simulink model "CEN598_HW2"  (R2015b)
settings: Solver=FixedStepDiscrete  SolverMode=SingleTasking  StartTime=0.0  StopTime=2.5e-6  RelTol=1e-3
libraries: shlslibv1 x212
(part 1 of 2)
settings Model: synDspstartup=OK  Creator=amitra5  LastModifiedBy=sjparekh
settings DataIOCC: SaveFormat=Array  SaveOutput=off  SignalLogging=off  SaveTime=off
settings OptimizationCC: DefaultParameterBehavior=Inlined
settings DebuggingCC: AlgebraicLoopMsg=error  SolverPrmCheckMsg=warning  InheritedTsInSrcMsg=none
settings HardwareCC: ProdBitPerPointer=32  ProdLargestAtomicFloat=None  ProdIntDivRoundTo=Undefined  ProdEndianess=Unspecified  ProdWordSize=32  ProdHWDeviceType=32-bit Generic
settings GRTTargetCC: GeneratePreprocessorConditionals=Disable all
settings ConfigComp: CovModelRefEnable=Off  CovSFcnEnable=off

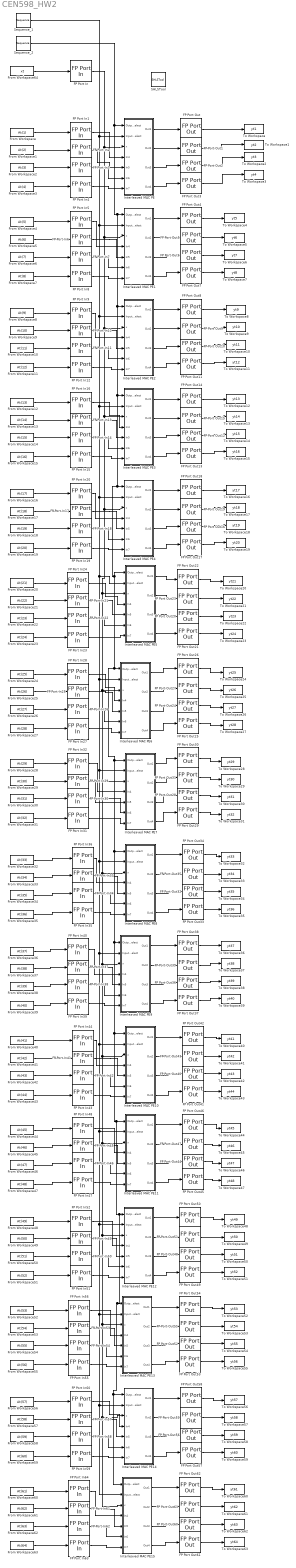
== system CEN598_HW2 ==
  FP Port In{,1..64} (65 alike) : shlslibv1/Floating Point/FP Port In  synBlockType=custom  synLatency=1  syn_exp_wl=11  syn_frac_wl=52  syn_out_st=1/284.04e6  syn_capture=on  syn_register=on  syn_opt_ports=off
  FP Port Out{,1..63} (64 alike) : shlslibv1/Floating Point/FP Port Out  synBlockType=custom  synLatency=1  syn_exp_wl=11  syn_frac_wl=52  syn_capture=on  syn_register=on
  From Workspace : FromWorkspace  VariableName=At(1)  Interpolate=off  OutputAfterFinalValue=Holding final value
  From Workspace1 : FromWorkspace  VariableName=At(2)  Interpolate=off  OutputAfterFinalValue=Holding final value
  From Workspace10 : FromWorkspace  VariableName=At(11)  Interpolate=off  OutputAfterFinalValue=Holding final value
  From Workspace11 : FromWorkspace  VariableName=At(12)  Interpolate=off  OutputAfterFinalValue=Holding final value
  From Workspace12 : FromWorkspace  VariableName=At(13)  Interpolate=off  OutputAfterFinalValue=Holding final value
  From Workspace13 : FromWorkspace  VariableName=At(14)  Interpolate=off  OutputAfterFinalValue=Holding final value
  From Workspace14 : FromWorkspace  VariableName=At(15)  Interpolate=off  OutputAfterFinalValue=Holding final value
  From Workspace15 : FromWorkspace  VariableName=At(16)  Interpolate=off  OutputAfterFinalValue=Holding final value
  From Workspace16 : FromWorkspace  VariableName=At(17)  Interpolate=off  OutputAfterFinalValue=Holding final value
  From Workspace17 : FromWorkspace  VariableName=At(18)  Interpolate=off  OutputAfterFinalValue=Holding final value
  From Workspace18 : FromWorkspace  VariableName=At(19)  Interpolate=off  OutputAfterFinalValue=Holding final value
  From Workspace19 : FromWorkspace  VariableName=At(20)  Interpolate=off  OutputAfterFinalValue=Holding final value
  From Workspace2 : FromWorkspace  VariableName=At(3)  Interpolate=off  OutputAfterFinalValue=Holding final value
  From Workspace20 : FromWorkspace  VariableName=At(21)  Interpolate=off  OutputAfterFinalValue=Holding final value
  From Workspace21 : FromWorkspace  VariableName=At(22)  Interpolate=off  OutputAfterFinalValue=Holding final value
  From Workspace22 : FromWorkspace  VariableName=At(23)  Interpolate=off  OutputAfterFinalValue=Holding final value
  From Workspace23 : FromWorkspace  VariableName=At(24)  Interpolate=off  OutputAfterFinalValue=Holding final value
  From Workspace24 : FromWorkspace  VariableName=At(25)  Interpolate=off  OutputAfterFinalValue=Holding final value
  From Workspace25 : FromWorkspace  VariableName=At(26)  Interpolate=off  OutputAfterFinalValue=Holding final value
  From Workspace26 : FromWorkspace  VariableName=At(27)  Interpolate=off  OutputAfterFinalValue=Holding final value
  From Workspace27 : FromWorkspace  VariableName=At(28)  Interpolate=off  OutputAfterFinalValue=Holding final value
  From Workspace28 : FromWorkspace  VariableName=At(29)  Interpolate=off  OutputAfterFinalValue=Holding final value
  From Workspace29 : FromWorkspace  VariableName=At(30)  Interpolate=off  OutputAfterFinalValue=Holding final value
  From Workspace3 : FromWorkspace  VariableName=At(4)  Interpolate=off  OutputAfterFinalValue=Holding final value
  From Workspace30 : FromWorkspace  VariableName=At(31)  Interpolate=off  OutputAfterFinalValue=Holding final value
  From Workspace31 : FromWorkspace  VariableName=At(32)  Interpolate=off  OutputAfterFinalValue=Holding final value
  From Workspace32 : FromWorkspace  VariableName=At(33)  Interpolate=off  OutputAfterFinalValue=Holding final value
  From Workspace33 : FromWorkspace  VariableName=At(34)  Interpolate=off  OutputAfterFinalValue=Holding final value
  From Workspace34 : FromWorkspace  VariableName=At(35)  Interpolate=off  OutputAfterFinalValue=Holding final value
  From Workspace35 : FromWorkspace  VariableName=At(36)  Interpolate=off  OutputAfterFinalValue=Holding final value
  From Workspace36 : FromWorkspace  VariableName=At(37)  Interpolate=off  OutputAfterFinalValue=Holding final value
  From Workspace37 : FromWorkspace  VariableName=At(38)  Interpolate=off  OutputAfterFinalValue=Holding final value
  From Workspace38 : FromWorkspace  VariableName=At(39)  Interpolate=off  OutputAfterFinalValue=Holding final value
  From Workspace39 : FromWorkspace  VariableName=At(40)  Interpolate=off  OutputAfterFinalValue=Holding final value
  From Workspace4 : FromWorkspace  VariableName=At(5)  Interpolate=off  OutputAfterFinalValue=Holding final value
  From Workspace40 : FromWorkspace  VariableName=At(41)  Interpolate=off  OutputAfterFinalValue=Holding final value
  From Workspace41 : FromWorkspace  VariableName=At(42)  Interpolate=off  OutputAfterFinalValue=Holding final value
  From Workspace42 : FromWorkspace  VariableName=At(43)  Interpolate=off  OutputAfterFinalValue=Holding final value
  From Workspace43 : FromWorkspace  VariableName=At(44)  Interpolate=off  OutputAfterFinalValue=Holding final value
  From Workspace44 : FromWorkspace  VariableName=At(45)  Interpolate=off  OutputAfterFinalValue=Holding final value
  From Workspace45 : FromWorkspace  VariableName=At(46)  Interpolate=off  OutputAfterFinalValue=Holding final value
  From Workspace46 : FromWorkspace  VariableName=At(47)  Interpolate=off  OutputAfterFinalValue=Holding final value
  From Workspace47 : FromWorkspace  VariableName=At(48)  Interpolate=off  OutputAfterFinalValue=Holding final value
  From Workspace48 : FromWorkspace  VariableName=At(49)  Interpolate=off  OutputAfterFinalValue=Holding final value
  From Workspace49 : FromWorkspace  VariableName=At(50)  Interpolate=off  OutputAfterFinalValue=Holding final value
  From Workspace5 : FromWorkspace  VariableName=At(6)  Interpolate=off  OutputAfterFinalValue=Holding final value
  From Workspace50 : FromWorkspace  VariableName=At(51)  Interpolate=off  OutputAfterFinalValue=Holding final value
  From Workspace51 : FromWorkspace  VariableName=At(52)  Interpolate=off  OutputAfterFinalValue=Holding final value
  From Workspace52 : FromWorkspace  VariableName=At(53)  Interpolate=off  OutputAfterFinalValue=Holding final value
  From Workspace53 : FromWorkspace  VariableName=At(54)  Interpolate=off  OutputAfterFinalValue=Holding final value
  From Workspace54 : FromWorkspace  VariableName=At(55)  Interpolate=off  OutputAfterFinalValue=Holding final value
  From Workspace55 : FromWorkspace  VariableName=At(56)  Interpolate=off  OutputAfterFinalValue=Holding final value
  From Workspace56 : FromWorkspace  VariableName=At(57)  Interpolate=off  OutputAfterFinalValue=Holding final value
  From Workspace57 : FromWorkspace  VariableName=At(58)  Interpolate=off  OutputAfterFinalValue=Holding final value
  From Workspace58 : FromWorkspace  VariableName=At(59)  Interpolate=off  OutputAfterFinalValue=Holding final value
  From Workspace59 : FromWorkspace  VariableName=At(60)  Interpolate=off  OutputAfterFinalValue=Holding final value
  From Workspace6 : FromWorkspace  VariableName=At(7)  Interpolate=off  OutputAfterFinalValue=Holding final value
  From Workspace60 : FromWorkspace  VariableName=At(61)  Interpolate=off  OutputAfterFinalValue=Holding final value
  From Workspace61 : FromWorkspace  VariableName=At(62)  Interpolate=off  OutputAfterFinalValue=Holding final value
  From Workspace62 : FromWorkspace  VariableName=At(63)  Interpolate=off  OutputAfterFinalValue=Holding final value
  From Workspace63 : FromWorkspace  VariableName=At(64)  Interpolate=off  OutputAfterFinalValue=Holding final value
  From Workspace64 : FromWorkspace  VariableName=xt  Interpolate=off  OutputAfterFinalValue=Holding final value
  From Workspace7 : FromWorkspace  VariableName=At(8)  Interpolate=off  OutputAfterFinalValue=Holding final value
  From Workspace8 : FromWorkspace  VariableName=At(9)  Interpolate=off  OutputAfterFinalValue=Holding final value
  From Workspace9 : FromWorkspace  VariableName=At(10)  Interpolate=off  OutputAfterFinalValue=Holding final value
  Interleaved MAC PE : Subsystem
  Interleaved MAC PE1 : Subsystem
  Interleaved MAC PE10 : Subsystem
  Interleaved MAC PE11 : Subsystem
  Interleaved MAC PE12 : Subsystem
  Interleaved MAC PE13 : Subsystem
  Interleaved MAC PE14 : Subsystem
  Interleaved MAC PE15 : Subsystem
  Interleaved MAC PE2 : Subsystem
  Interleaved MAC PE3 : Subsystem
  Interleaved MAC PE4 : Subsystem
  Interleaved MAC PE5 : Subsystem
  Interleaved MAC PE6 : Subsystem
  Interleaved MAC PE7 : Subsystem
  Interleaved MAC PE8 : Subsystem
  Interleaved MAC PE9 : Subsystem
  SHLSTool : shlslibv1/SHLSTool  synBlockType=tool  syn_dsp_mode=FPGA
  Sequence_1 : shlslibv1/Sources/Sequence  syn_seq_vec=[0 1 2 3 0 0 0 0 0]  syn_seq_wl=2  syn_seq_fl=0  syn_seq_dt=unsigned  syn_rst_port=off  syn_en_port=off  syn_seq_st=1/284.04e6  synBlockType=custom  synLatency=1
  Sequence_2 : shlslibv1/Sources/Sequence  syn_seq_vec=[0 0 0 0 1 2 3 0 0]  syn_seq_wl=2  syn_seq_fl=0  syn_seq_dt=unsigned  syn_rst_port=off  syn_en_port=off  syn_seq_st=1/284.04e6  synBlockType=custom  synLatency=1
  To Workspace : ToWorkspace  VariableName=yt1  SaveFormat=Structure With Time  SampleTime=-1
      settings: Save2DSignal=2-D array (concatenate along first dimension)
  To Workspace1 : ToWorkspace  VariableName=yt2  SaveFormat=Structure With Time  SampleTime=-1
      settings: Save2DSignal=2-D array (concatenate along first dimension)
  To Workspace10 : ToWorkspace  VariableName=yt11  SaveFormat=Structure With Time  SampleTime=-1
      settings: Save2DSignal=2-D array (concatenate along first dimension)
  To Workspace11 : ToWorkspace  VariableName=yt12  SaveFormat=Structure With Time  SampleTime=-1
  To Workspace12 : ToWorkspace  VariableName=yt13  SaveFormat=Structure With Time  SampleTime=-1
      settings: Save2DSignal=2-D array (concatenate along first dimension)
  To Workspace13 : ToWorkspace  VariableName=yt14  SaveFormat=Structure With Time  SampleTime=-1
      settings: Save2DSignal=2-D array (concatenate along first dimension)
  To Workspace14 : ToWorkspace  VariableName=yt15  SaveFormat=Structure With Time  SampleTime=-1
      settings: Save2DSignal=2-D array (concatenate along first dimension)
  To Workspace15 : ToWorkspace  VariableName=yt16  SaveFormat=Structure With Time  SampleTime=-1
  To Workspace16 : ToWorkspace  VariableName=yt17  SaveFormat=Structure With Time  SampleTime=-1
      settings: Save2DSignal=2-D array (concatenate along first dimension)
  To Workspace17 : ToWorkspace  VariableName=yt18  SaveFormat=Structure With Time  SampleTime=-1
      settings: Save2DSignal=2-D array (concatenate along first dimension)
  To Workspace18 : ToWorkspace  VariableName=yt19  SaveFormat=Structure With Time  SampleTime=-1
      settings: Save2DSignal=2-D array (concatenate along first dimension)
  To Workspace19 : ToWorkspace  VariableName=yt20  SaveFormat=Structure With Time  SampleTime=-1
  To Workspace2 : ToWorkspace  VariableName=yt3  SaveFormat=Structure With Time  SampleTime=-1
      settings: Save2DSignal=2-D array (concatenate along first dimension)
  To Workspace20 : ToWorkspace  VariableName=yt21  SaveFormat=Structure With Time  SampleTime=-1
      settings: Save2DSignal=2-D array (concatenate along first dimension)
  To Workspace21 : ToWorkspace  VariableName=yt22  SaveFormat=Structure With Time  SampleTime=-1
      settings: Save2DSignal=2-D array (concatenate along first dimension)
  To Workspace22 : ToWorkspace  VariableName=yt23  SaveFormat=Structure With Time  SampleTime=-1
      settings: Save2DSignal=2-D array (concatenate along first dimension)
  To Workspace23 : ToWorkspace  VariableName=yt24  SaveFormat=Structure With Time  SampleTime=-1
  To Workspace24 : ToWorkspace  VariableName=yt25  SaveFormat=Structure With Time  SampleTime=-1
      settings: Save2DSignal=2-D array (concatenate along first dimension)
  To Workspace25 : ToWorkspace  VariableName=yt26  SaveFormat=Structure With Time  SampleTime=-1
      settings: Save2DSignal=2-D array (concatenate along first dimension)
  To Workspace26 : ToWorkspace  VariableName=yt27  SaveFormat=Structure With Time  SampleTime=-1
      settings: Save2DSignal=2-D array (concatenate along first dimension)
  To Workspace27 : ToWorkspace  VariableName=yt28  SaveFormat=Structure With Time  SampleTime=-1
  To Workspace28 : ToWorkspace  VariableName=yt29  SaveFormat=Structure With Time  SampleTime=-1
      settings: Save2DSignal=2-D array (concatenate along first dimension)
  To Workspace29 : ToWorkspace  VariableName=yt30  SaveFormat=Structure With Time  SampleTime=-1
      settings: Save2DSignal=2-D array (concatenate along first dimension)
  To Workspace3 : ToWorkspace  VariableName=yt4  SaveFormat=Structure With Time  SampleTime=-1
  To Workspace30 : ToWorkspace  VariableName=yt31  SaveFormat=Structure With Time  SampleTime=-1
      settings: Save2DSignal=2-D array (concatenate along first dimension)
  To Workspace31 : ToWorkspace  VariableName=yt32  SaveFormat=Structure With Time  SampleTime=-1
  To Workspace32 : ToWorkspace  VariableName=yt33  SaveFormat=Structure With Time  SampleTime=-1
      settings: Save2DSignal=2-D array (concatenate along first dimension)
  To Workspace33 : ToWorkspace  VariableName=yt34  SaveFormat=Structure With Time  SampleTime=-1
      settings: Save2DSignal=2-D array (concatenate along first dimension)
  To Workspace34 : ToWorkspace  VariableName=yt35  SaveFormat=Structure With Time  SampleTime=-1
      settings: Save2DSignal=2-D array (concatenate along first dimension)
  To Workspace35 : ToWorkspace  VariableName=yt36  SaveFormat=Structure With Time  SampleTime=-1
  To Workspace36 : ToWorkspace  VariableName=yt37  SaveFormat=Structure With Time  SampleTime=-1
      settings: Save2DSignal=2-D array (concatenate along first dimension)
  To Workspace37 : ToWorkspace  VariableName=yt38  SaveFormat=Structure With Time  SampleTime=-1
      settings: Save2DSignal=2-D array (concatenate along first dimension)
  To Workspace38 : ToWorkspace  VariableName=yt39  SaveFormat=Structure With Time  SampleTime=-1
      settings: Save2DSignal=2-D array (concatenate along first dimension)
  To Workspace39 : ToWorkspace  VariableName=yt40  SaveFormat=Structure With Time  SampleTime=-1
  To Workspace4 : ToWorkspace  VariableName=yt5  SaveFormat=Structure With Time  SampleTime=-1
      settings: Save2DSignal=2-D array (concatenate along first dimension)
  To Workspace40 : ToWorkspace  VariableName=yt41  SaveFormat=Structure With Time  SampleTime=-1
      settings: Save2DSignal=2-D array (concatenate along first dimension)
  To Workspace41 : ToWorkspace  VariableName=yt42  SaveFormat=Structure With Time  SampleTime=-1
      settings: Save2DSignal=2-D array (concatenate along first dimension)
  To Workspace42 : ToWorkspace  VariableName=yt43  SaveFormat=Structure With Time  SampleTime=-1
      settings: Save2DSignal=2-D array (concatenate along first dimension)
  To Workspace43 : ToWorkspace  VariableName=yt44  SaveFormat=Structure With Time  SampleTime=-1
  To Workspace44 : ToWorkspace  VariableName=yt45  SaveFormat=Structure With Time  SampleTime=-1
      settings: Save2DSignal=2-D array (concatenate along first dimension)
  To Workspace45 : ToWorkspace  VariableName=yt46  SaveFormat=Structure With Time  SampleTime=-1
      settings: Save2DSignal=2-D array (concatenate along first dimension)
  To Workspace46 : ToWorkspace  VariableName=yt47  SaveFormat=Structure With Time  SampleTime=-1
      settings: Save2DSignal=2-D array (concatenate along first dimension)
  To Workspace47 : ToWorkspace  VariableName=yt48  SaveFormat=Structure With Time  SampleTime=-1
  To Workspace48 : ToWorkspace  VariableName=yt49  SaveFormat=Structure With Time  SampleTime=-1
      settings: Save2DSignal=2-D array (concatenate along first dimension)
  To Workspace49 : ToWorkspace  VariableName=yt50  SaveFormat=Structure With Time  SampleTime=-1
      settings: Save2DSignal=2-D array (concatenate along first dimension)
  To Workspace5 : ToWorkspace  VariableName=yt6  SaveFormat=Structure With Time  SampleTime=-1
      settings: Save2DSignal=2-D array (concatenate along first dimension)
  To Workspace50 : ToWorkspace  VariableName=yt51  SaveFormat=Structure With Time  SampleTime=-1
      settings: Save2DSignal=2-D array (concatenate along first dimension)
  To Workspace51 : ToWorkspace  VariableName=yt52  SaveFormat=Structure With Time  SampleTime=-1
  To Workspace52 : ToWorkspace  VariableName=yt53  SaveFormat=Structure With Time  SampleTime=-1
      settings: Save2DSignal=2-D array (concatenate along first dimension)
  To Workspace53 : ToWorkspace  VariableName=yt54  SaveFormat=Structure With Time  SampleTime=-1
      settings: Save2DSignal=2-D array (concatenate along first dimension)
  To Workspace54 : ToWorkspace  VariableName=yt55  SaveFormat=Structure With Time  SampleTime=-1
      settings: Save2DSignal=2-D array (concatenate along first dimension)
  To Workspace55 : ToWorkspace  VariableName=yt56  SaveFormat=Structure With Time  SampleTime=-1
  To Workspace56 : ToWorkspace  VariableName=yt57  SaveFormat=Structure With Time  SampleTime=-1
      settings: Save2DSignal=2-D array (concatenate along first dimension)
  To Workspace57 : ToWorkspace  VariableName=yt58  SaveFormat=Structure With Time  SampleTime=-1
      settings: Save2DSignal=2-D array (concatenate along first dimension)
  To Workspace58 : ToWorkspace  VariableName=yt59  SaveFormat=Structure With Time  SampleTime=-1
      settings: Save2DSignal=2-D array (concatenate along first dimension)
  To Workspace59 : ToWorkspace  VariableName=yt60  SaveFormat=Structure With Time  SampleTime=-1
  To Workspace6 : ToWorkspace  VariableName=yt7  SaveFormat=Structure With Time  SampleTime=-1
      settings: Save2DSignal=2-D array (concatenate along first dimension)
  To Workspace60 : ToWorkspace  VariableName=yt61  SaveFormat=Structure With Time  SampleTime=-1
      settings: Save2DSignal=2-D array (concatenate along first dimension)
  To Workspace61 : ToWorkspace  VariableName=yt62  SaveFormat=Structure With Time  SampleTime=-1
      settings: Save2DSignal=2-D array (concatenate along first dimension)
  To Workspace62 : ToWorkspace  VariableName=yt63  SaveFormat=Structure With Time  SampleTime=-1
      settings: Save2DSignal=2-D array (concatenate along first dimension)
  To Workspace63 : ToWorkspace  VariableName=yt64  SaveFormat=Structure With Time  SampleTime=-1
  To Workspace7 : ToWorkspace  VariableName=yt8  SaveFormat=Structure With Time  SampleTime=-1
  To Workspace8 : ToWorkspace  VariableName=yt9  SaveFormat=Structure With Time  SampleTime=-1
      settings: Save2DSignal=2-D array (concatenate along first dimension)
  To Workspace9 : ToWorkspace  VariableName=yt10  SaveFormat=Structure With Time  SampleTime=-1
      settings: Save2DSignal=2-D array (concatenate along first dimension)
  wires:
  From Workspace/1 -> FP Port In1/1
  From Workspace1/1 -> FP Port In2/1
  From Workspace2/1 -> FP Port In3/1
  From Workspace3/1 -> FP Port In4/1
  FP Port Out2/1 -> To Workspace2/1
  FP Port Out3/1 -> To Workspace3/1
  FP Port Out4/1 -> To Workspace4/1
  FP Port Out5/1 -> To Workspace5/1
  FP Port Out6/1 -> To Workspace6/1
  FP Port Out7/1 -> To Workspace7/1
  FP Port Out8/1 -> To Workspace8/1
  FP Port Out9/1 -> To Workspace9/1
  FP Port Out10/1 -> To Workspace10/1
  FP Port Out11/1 -> To Workspace11/1
  FP Port Out14/1 -> To Workspace12/1
  FP Port Out15/1 -> To Workspace13/1
  FP Port Out12/1 -> To Workspace14/1
  FP Port Out13/1 -> To Workspace15/1
  FP Port Out18/1 -> To Workspace16/1
  FP Port Out19/1 -> To Workspace17/1
  FP Port Out16/1 -> To Workspace18/1
  FP Port Out17/1 -> To Workspace19/1
  FP Port Out22/1 -> To Workspace20/1
  FP Port Out23/1 -> To Workspace21/1
  FP Port Out20/1 -> To Workspace22/1
  FP Port Out21/1 -> To Workspace23/1
  FP Port Out26/1 -> To Workspace24/1
  FP Port Out27/1 -> To Workspace25/1
  FP Port Out24/1 -> To Workspace26/1
  FP Port Out25/1 -> To Workspace27/1
  FP Port Out30/1 -> To Workspace28/1
  FP Port Out31/1 -> To Workspace29/1
  FP Port Out28/1 -> To Workspace30/1
  FP Port Out29/1 -> To Workspace31/1
  FP Port Out34/1 -> To Workspace32/1
  FP Port Out35/1 -> To Workspace33/1
  FP Port Out32/1 -> To Workspace34/1
  FP Port Out33/1 -> To Workspace35/1
  FP Port Out38/1 -> To Workspace36/1
  FP Port Out39/1 -> To Workspace37/1
  FP Port Out36/1 -> To Workspace38/1
  FP Port Out37/1 -> To Workspace39/1
  FP Port Out42/1 -> To Workspace40/1
  FP Port Out43/1 -> To Workspace41/1
  FP Port Out40/1 -> To Workspace42/1
  FP Port Out41/1 -> To Workspace43/1
  FP Port Out46/1 -> To Workspace44/1
  FP Port Out47/1 -> To Workspace45/1
  FP Port Out44/1 -> To Workspace46/1
  FP Port Out45/1 -> To Workspace47/1
  FP Port Out50/1 -> To Workspace48/1
  FP Port Out51/1 -> To Workspace49/1
  FP Port Out48/1 -> To Workspace50/1
  FP Port Out49/1 -> To Workspace51/1
  FP Port Out54/1 -> To Workspace52/1
  FP Port Out55/1 -> To Workspace53/1
  FP Port Out52/1 -> To Workspace54/1
  FP Port Out53/1 -> To Workspace55/1
  FP Port Out58/1 -> To Workspace56/1
  FP Port Out59/1 -> To Workspace57/1
  FP Port Out56/1 -> To Workspace58/1
  FP Port Out57/1 -> To Workspace59/1
  FP Port Out62/1 -> To Workspace60/1
  FP Port Out63/1 -> To Workspace61/1
  FP Port Out60/1 -> To Workspace62/1
  FP Port Out61/1 -> To Workspace63/1
  From Workspace4/1 -> FP Port In5/1
  From Workspace5/1 -> FP Port In6/1
  From Workspace6/1 -> FP Port In7/1
  From Workspace7/1 -> FP Port In8/1
  From Workspace8/1 -> FP Port In9/1
  From Workspace9/1 -> FP Port In10/1
  From Workspace10/1 -> FP Port In11/1
  From Workspace11/1 -> FP Port In12/1
  From Workspace12/1 -> FP Port In16/1
  From Workspace13/1 -> FP Port In13/1
  From Workspace14/1 -> FP Port In14/1
  From Workspace15/1 -> FP Port In15/1
  From Workspace16/1 -> FP Port In20/1
  From Workspace17/1 -> FP Port In17/1
  From Workspace18/1 -> FP Port In18/1
  From Workspace19/1 -> FP Port In19/1
  From Workspace20/1 -> FP Port In24/1
  From Workspace21/1 -> FP Port In21/1
  From Workspace22/1 -> FP Port In22/1
  From Workspace23/1 -> FP Port In23/1
  From Workspace24/1 -> FP Port In28/1
  From Workspace25/1 -> FP Port In25/1
  From Workspace26/1 -> FP Port In26/1
  From Workspace27/1 -> FP Port In27/1
  From Workspace28/1 -> FP Port In32/1
  From Workspace29/1 -> FP Port In29/1
  From Workspace30/1 -> FP Port In30/1
  From Workspace31/1 -> FP Port In31/1
  From Workspace32/1 -> FP Port In36/1
  From Workspace33/1 -> FP Port In33/1
  From Workspace34/1 -> FP Port In34/1
  From Workspace35/1 -> FP Port In35/1
  From Workspace36/1 -> FP Port In40/1
  From Workspace37/1 -> FP Port In37/1
  From Workspace38/1 -> FP Port In38/1
  From Workspace39/1 -> FP Port In39/1
  From Workspace40/1 -> FP Port In44/1
  From Workspace41/1 -> FP Port In41/1
  From Workspace42/1 -> FP Port In42/1
  From Workspace43/1 -> FP Port In43/1
  From Workspace44/1 -> FP Port In48/1
  From Workspace45/1 -> FP Port In45/1
  From Workspace46/1 -> FP Port In46/1
  From Workspace47/1 -> FP Port In47/1
  From Workspace48/1 -> FP Port In52/1
  From Workspace49/1 -> FP Port In49/1
  From Workspace50/1 -> FP Port In50/1
  From Workspace51/1 -> FP Port In51/1
  From Workspace52/1 -> FP Port In56/1
  From Workspace53/1 -> FP Port In53/1
  From Workspace54/1 -> FP Port In54/1
  From Workspace55/1 -> FP Port In55/1
  From Workspace56/1 -> FP Port In60/1
  From Workspace57/1 -> FP Port In57/1
  From Workspace58/1 -> FP Port In58/1
  From Workspace59/1 -> FP Port In59/1
  From Workspace60/1 -> FP Port In64/1
  From Workspace61/1 -> FP Port In61/1
  From Workspace62/1 -> FP Port In62/1
  From Workspace63/1 -> FP Port In63/1
  From Workspace64/1 -> FP Port In/1
  FP Port Out/1 -> To Workspace/1
  Interleaved MAC PE/1(Out1) -> FP Port Out/1
  FP Port In4/1 -> Interleaved MAC PE/7(In7)
  FP Port In3/1 -> Interleaved MAC PE/6(In6)
  FP Port In2/1 -> Interleaved MAC PE/5(In5)
  FP Port In1/1 -> Interleaved MAC PE/4(In4)
  FP Port Out1/1 -> To Workspace1/1
  Interleaved MAC PE/2(Out2) -> FP Port Out1/1
  Interleaved MAC PE/3(Out3) -> FP Port Out2/1
  Interleaved MAC PE/4(Out4) -> FP Port Out3/1
  Interleaved MAC PE1/1(Out1) -> FP Port Out4/1
  FP Port In8/1 -> Interleaved MAC PE1/7(In7)
  FP Port In7/1 -> Interleaved MAC PE1/6(In6)
  FP Port In6/1 -> Interleaved MAC PE1/5(In5)
  FP Port In5/1 -> Interleaved MAC PE1/4(In4)
  Interleaved MAC PE1/2(Out2) -> FP Port Out5/1
  Interleaved MAC PE1/3(Out3) -> FP Port Out6/1
  Interleaved MAC PE1/4(Out4) -> FP Port Out7/1
  Interleaved MAC PE2/1(Out1) -> FP Port Out8/1
  FP Port In12/1 -> Interleaved MAC PE2/7(In7)
  FP Port In11/1 -> Interleaved MAC PE2/6(In6)
  FP Port In10/1 -> Interleaved MAC PE2/5(In5)
  FP Port In9/1 -> Interleaved MAC PE2/4(In4)
  Interleaved MAC PE2/2(Out2) -> FP Port Out9/1
  Interleaved MAC PE2/3(Out3) -> FP Port Out10/1
  Interleaved MAC PE2/4(Out4) -> FP Port Out11/1
  Interleaved MAC PE3/1(Out1) -> FP Port Out14/1
  FP Port In15/1 -> Interleaved MAC PE3/7(In7)
  FP Port In14/1 -> Interleaved MAC PE3/6(In6)
  FP Port In13/1 -> Interleaved MAC PE3/5(In5)
  FP Port In16/1 -> Interleaved MAC PE3/4(In4)
  Interleaved MAC PE3/2(Out2) -> FP Port Out15/1
  Interleaved MAC PE3/3(Out3) -> FP Port Out12/1
  Interleaved MAC PE3/4(Out4) -> FP Port Out13/1
  Interleaved MAC PE4/1(Out1) -> FP Port Out18/1
  FP Port In19/1 -> Interleaved MAC PE4/7(In7)
  FP Port In18/1 -> Interleaved MAC PE4/6(In6)
  FP Port In17/1 -> Interleaved MAC PE4/5(In5)
  FP Port In20/1 -> Interleaved MAC PE4/4(In4)
  Interleaved MAC PE4/2(Out2) -> FP Port Out19/1
  Interleaved MAC PE4/3(Out3) -> FP Port Out16/1
  Interleaved MAC PE4/4(Out4) -> FP Port Out17/1
  Interleaved MAC PE5/1(Out1) -> FP Port Out22/1
  FP Port In23/1 -> Interleaved MAC PE5/7(In7)
  FP Port In22/1 -> Interleaved MAC PE5/6(In6)
  FP Port In21/1 -> Interleaved MAC PE5/5(In5)
  FP Port In24/1 -> Interleaved MAC PE5/4(In4)
  Interleaved MAC PE5/2(Out2) -> FP Port Out23/1
  Interleaved MAC PE5/3(Out3) -> FP Port Out20/1
  Interleaved MAC PE5/4(Out4) -> FP Port Out21/1
  Interleaved MAC PE6/1(Out1) -> FP Port Out26/1
  FP Port In27/1 -> Interleaved MAC PE6/7(In7)
  FP Port In26/1 -> Interleaved MAC PE6/6(In6)
  FP Port In25/1 -> Interleaved MAC PE6/5(In5)
  FP Port In28/1 -> Interleaved MAC PE6/4(In4)
  Interleaved MAC PE6/2(Out2) -> FP Port Out27/1
  Interleaved MAC PE6/3(Out3) -> FP Port Out24/1
  Interleaved MAC PE6/4(Out4) -> FP Port Out25/1
  Interleaved MAC PE7/1(Out1) -> FP Port Out30/1
  FP Port In31/1 -> Interleaved MAC PE7/7(In7)
  FP Port In30/1 -> Interleaved MAC PE7/6(In6)
  FP Port In29/1 -> Interleaved MAC PE7/5(In5)
  FP Port In32/1 -> Interleaved MAC PE7/4(In4)
  Interleaved MAC PE7/2(Out2) -> FP Port Out31/1
  Interleaved MAC PE7/3(Out3) -> FP Port Out28/1
  Interleaved MAC PE7/4(Out4) -> FP Port Out29/1
  Interleaved MAC PE8/1(Out1) -> FP Port Out34/1
  FP Port In35/1 -> Interleaved MAC PE8/7(In7)
  FP Port In34/1 -> Interleaved MAC PE8/6(In6)
  FP Port In33/1 -> Interleaved MAC PE8/5(In5)
  FP Port In36/1 -> Interleaved MAC PE8/4(In4)
  Interleaved MAC PE8/2(Out2) -> FP Port Out35/1
  Interleaved MAC PE8/3(Out3) -> FP Port Out32/1
  Interleaved MAC PE8/4(Out4) -> FP Port Out33/1
  Interleaved MAC PE9/1(Out1) -> FP Port Out38/1
  FP Port In39/1 -> Interleaved MAC PE9/7(In7)
  FP Port In38/1 -> Interleaved MAC PE9/6(In6)
  FP Port In37/1 -> Interleaved MAC PE9/5(In5)
  FP Port In40/1 -> Interleaved MAC PE9/4(In4)
  Interleaved MAC PE9/2(Out2) -> FP Port Out39/1
  Interleaved MAC PE9/3(Out3) -> FP Port Out36/1
  Interleaved MAC PE9/4(Out4) -> FP Port Out37/1
  Interleaved MAC PE10/1(Out1) -> FP Port Out42/1
  FP Port In43/1 -> Interleaved MAC PE10/7(In7)
  FP Port In42/1 -> Interleaved MAC PE10/6(In6)
  FP Port In41/1 -> Interleaved MAC PE10/5(In5)
  FP Port In44/1 -> Interleaved MAC PE10/4(In4)
  Interleaved MAC PE10/2(Out2) -> FP Port Out43/1
  Interleaved MAC PE10/3(Out3) -> FP Port Out40/1
  Interleaved MAC PE10/4(Out4) -> FP Port Out41/1
  Interleaved MAC PE11/1(Out1) -> FP Port Out46/1
  FP Port In47/1 -> Interleaved MAC PE11/7(In7)
  FP Port In46/1 -> Interleaved MAC PE11/6(In6)
  FP Port In45/1 -> Interleaved MAC PE11/5(In5)
  FP Port In48/1 -> Interleaved MAC PE11/4(In4)
  Interleaved MAC PE11/2(Out2) -> FP Port Out47/1
  Interleaved MAC PE11/3(Out3) -> FP Port Out44/1
  Interleaved MAC PE11/4(Out4) -> FP Port Out45/1
  Interleaved MAC PE12/1(Out1) -> FP Port Out50/1
  FP Port In51/1 -> Interleaved MAC PE12/7(In7)
  FP Port In50/1 -> Interleaved MAC PE12/6(In6)
  FP Port In49/1 -> Interleaved MAC PE12/5(In5)
  FP Port In52/1 -> Interleaved MAC PE12/4(In4)
  Interleaved MAC PE12/2(Out2) -> FP Port Out51/1
  Interleaved MAC PE12/3(Out3) -> FP Port Out48/1
  Interleaved MAC PE12/4(Out4) -> FP Port Out49/1
  Interleaved MAC PE13/1(Out1) -> FP Port Out54/1
  FP Port In55/1 -> Interleaved MAC PE13/7(In7)
  FP Port In54/1 -> Interleaved MAC PE13/6(In6)
  FP Port In53/1 -> Interleaved MAC PE13/5(In5)
  FP Port In56/1 -> Interleaved MAC PE13/4(In4)
  Interleaved MAC PE13/2(Out2) -> FP Port Out55/1
  Interleaved MAC PE13/3(Out3) -> FP Port Out52/1
  Interleaved MAC PE13/4(Out4) -> FP Port Out53/1
  Interleaved MAC PE14/1(Out1) -> FP Port Out58/1
  FP Port In59/1 -> Interleaved MAC PE14/7(In7)
  FP Port In58/1 -> Interleaved MAC PE14/6(In6)
  FP Port In57/1 -> Interleaved MAC PE14/5(In5)
  FP Port In60/1 -> Interleaved MAC PE14/4(In4)
  Interleaved MAC PE14/2(Out2) -> FP Port Out59/1
  Interleaved MAC PE14/3(Out3) -> FP Port Out56/1
  Interleaved MAC PE14/4(Out4) -> FP Port Out57/1
  Interleaved MAC PE15/1(Out1) -> FP Port Out62/1
  FP Port In63/1 -> Interleaved MAC PE15/7(In7)
  FP Port In62/1 -> Interleaved MAC PE15/6(In6)
  FP Port In61/1 -> Interleaved MAC PE15/5(In5)
  FP Port In64/1 -> Interleaved MAC PE15/4(In4)
  Interleaved MAC PE15/2(Out2) -> FP Port Out63/1
  Interleaved MAC PE15/3(Out3) -> FP Port Out60/1
  Interleaved MAC PE15/4(Out4) -> FP Port Out61/1
  FP Port In/1 -> Interleaved MAC PE/3(x), Interleaved MAC PE1/3(x), Interleaved MAC PE2/3(x), Interleaved MAC PE4/3(x), Interleaved MAC PE6/3(x), Interleaved MAC PE7/3(x), Interleaved MAC PE8/3(x), Interleaved MAC PE9/3(x), Interleaved MAC PE10/3(x), Interleaved MAC PE11/3(x), Interleaved MAC PE12/3(x), Interleaved MAC PE13/3(x), Interleaved MAC PE14/3(x), Interleaved MAC PE15/3(x), Interleaved MAC PE5/3(x), Interleaved MAC PE3/3(x)
  Sequence_2/1 -> Interleaved MAC PE3/1(Output_Select), Interleaved MAC PE4/1(Output_Select), Interleaved MAC PE6/1(Output_Select), Interleaved MAC PE8/1(Output_Select), Interleaved MAC PE10/1(Output_Select), Interleaved MAC PE14/1(Output_Select), Interleaved MAC PE15/1(Output_Select), Interleaved MAC PE13/1(Output_Select), Interleaved MAC PE12/1(Output_Select), Interleaved MAC PE11/1(Output_Select), Interleaved MAC PE9/1(Output_Select), Interleaved MAC PE7/1(Output_Select), Interleaved MAC PE5/1(Output_Select), Interleaved MAC PE2/1(Output_Select), Interleaved MAC PE1/1(Output_Select), Interleaved MAC PE/1(Output_Select)
  Sequence_1/1 -> Interleaved MAC PE/2(Input_Select), Interleaved MAC PE3/2(Input_Select), Interleaved MAC PE4/2(Input_Select), Interleaved MAC PE5/2(Input_Select), Interleaved MAC PE6/2(Input_Select), Interleaved MAC PE7/2(Input_Select), Interleaved MAC PE15/2(Input_Select), Interleaved MAC PE14/2(Input_Select), Interleaved MAC PE13/2(Input_Select), Interleaved MAC PE12/2(Input_Select), Interleaved MAC PE11/2(Input_Select), Interleaved MAC PE10/2(Input_Select), Interleaved MAC PE9/2(Input_Select), Interleaved MAC PE8/2(Input_Select), Interleaved MAC PE2/2(Input_Select), Interleaved MAC PE1/2(Input_Select)

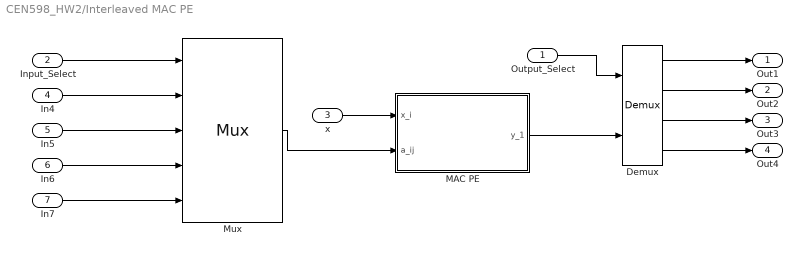
== system CEN598_HW2/Interleaved MAC PE ==
  Output_Select : Inport
  Input_Select : Inport  Port=2
  x : Inport  Port=3
  In4 : Inport  Port=4
  In5 : Inport  Port=5
  In6 : Inport  Port=6
  In7 : Inport  Port=7
  Demux : shlslibv1/Signal Operations/Demux  syn_out_nb=4  syn_out_latch=off  synBlockType=primitive  synLatency=0  synBlockId=18
  MAC PE : Subsystem
  Mux : shlslibv1/Signal Operations/Mux  syn_in_nb=4  syn_out_f=Full Precision  syn_out_wl=16  syn_out_fl=8  syn_out_dt=signed  syn_en_se=off  synBlockType=primitive  synLatency=0  synBlockId=16
  Out1 : Outport
  Out2 : Outport  Port=2
  Out3 : Outport  Port=3
  Out4 : Outport  Port=4
  wires:
  Demux/1 -> Out1/1
  Demux/2 -> Out2/1
  Demux/3 -> Out3/1
  Demux/4 -> Out4/1
  Output_Select/1 -> Demux/1
  Input_Select/1 -> Mux/1
  In4/1 -> Mux/2
  In5/1 -> Mux/3
  In6/1 -> Mux/4
  In7/1 -> Mux/5
  Mux/1 -> MAC PE/2(a_ij)
  x/1 -> MAC PE/1(x_i)
  MAC PE/1(y_1) -> Demux/2

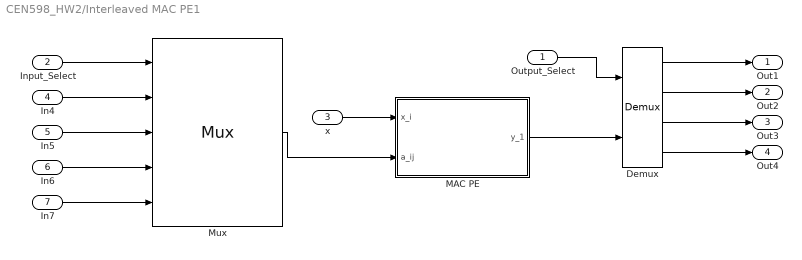
== system CEN598_HW2/Interleaved MAC PE1 ==
  Output_Select : Inport
  Input_Select : Inport  Port=2
  x : Inport  Port=3
  In4 : Inport  Port=4
  In5 : Inport  Port=5
  In6 : Inport  Port=6
  In7 : Inport  Port=7
  Demux : shlslibv1/Signal Operations/Demux  syn_out_nb=4  syn_out_latch=off  synBlockType=primitive  synLatency=0  synBlockId=18
  MAC PE : Subsystem
  Mux : shlslibv1/Signal Operations/Mux  syn_in_nb=4  syn_out_f=Full Precision  syn_out_wl=16  syn_out_fl=8  syn_out_dt=signed  syn_en_se=off  synBlockType=primitive  synLatency=0  synBlockId=16
  Out1 : Outport
  Out2 : Outport  Port=2
  Out3 : Outport  Port=3
  Out4 : Outport  Port=4
  wires:
  Demux/1 -> Out1/1
  Demux/2 -> Out2/1
  Demux/3 -> Out3/1
  Demux/4 -> Out4/1
  Output_Select/1 -> Demux/1
  Input_Select/1 -> Mux/1
  In4/1 -> Mux/2
  In5/1 -> Mux/3
  In6/1 -> Mux/4
  In7/1 -> Mux/5
  Mux/1 -> MAC PE/2(a_ij)
  x/1 -> MAC PE/1(x_i)
  MAC PE/1(y_1) -> Demux/2

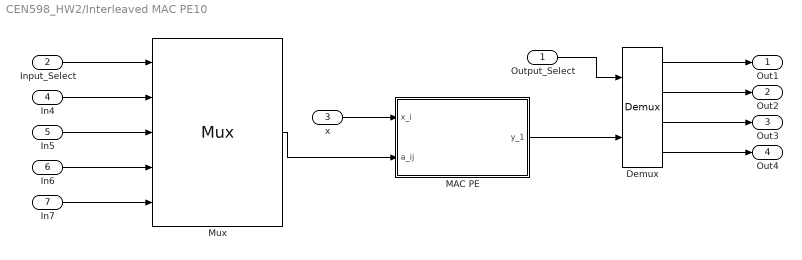
== system CEN598_HW2/Interleaved MAC PE10 ==
  Output_Select : Inport
  Input_Select : Inport  Port=2
  x : Inport  Port=3
  In4 : Inport  Port=4
  In5 : Inport  Port=5
  In6 : Inport  Port=6
  In7 : Inport  Port=7
  Demux : shlslibv1/Signal Operations/Demux  syn_out_nb=4  syn_out_latch=off  synBlockType=primitive  synLatency=0  synBlockId=18
  MAC PE : Subsystem
  Mux : shlslibv1/Signal Operations/Mux  syn_in_nb=4  syn_out_f=Full Precision  syn_out_wl=16  syn_out_fl=8  syn_out_dt=signed  syn_en_se=off  synBlockType=primitive  synLatency=0  synBlockId=16
  Out1 : Outport
  Out2 : Outport  Port=2
  Out3 : Outport  Port=3
  Out4 : Outport  Port=4
  wires:
  Demux/1 -> Out1/1
  Demux/2 -> Out2/1
  Demux/3 -> Out3/1
  Demux/4 -> Out4/1
  Output_Select/1 -> Demux/1
  Input_Select/1 -> Mux/1
  In4/1 -> Mux/2
  In5/1 -> Mux/3
  In6/1 -> Mux/4
  In7/1 -> Mux/5
  Mux/1 -> MAC PE/2(a_ij)
  x/1 -> MAC PE/1(x_i)
  MAC PE/1(y_1) -> Demux/2

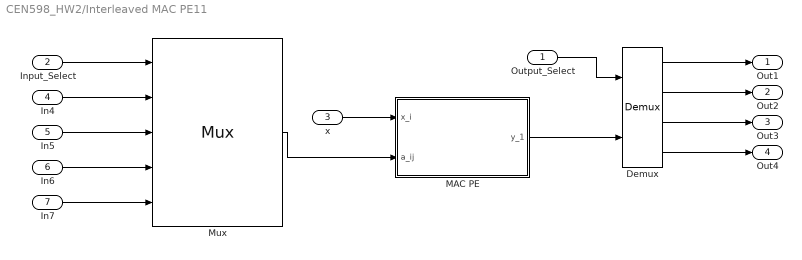
== system CEN598_HW2/Interleaved MAC PE11 ==
  Output_Select : Inport
  Input_Select : Inport  Port=2
  x : Inport  Port=3
  In4 : Inport  Port=4
  In5 : Inport  Port=5
  In6 : Inport  Port=6
  In7 : Inport  Port=7
  Demux : shlslibv1/Signal Operations/Demux  syn_out_nb=4  syn_out_latch=off  synBlockType=primitive  synLatency=0  synBlockId=18
  MAC PE : Subsystem
  Mux : shlslibv1/Signal Operations/Mux  syn_in_nb=4  syn_out_f=Full Precision  syn_out_wl=16  syn_out_fl=8  syn_out_dt=signed  syn_en_se=off  synBlockType=primitive  synLatency=0  synBlockId=16
  Out1 : Outport
  Out2 : Outport  Port=2
  Out3 : Outport  Port=3
  Out4 : Outport  Port=4
  wires:
  Demux/1 -> Out1/1
  Demux/2 -> Out2/1
  Demux/3 -> Out3/1
  Demux/4 -> Out4/1
  Output_Select/1 -> Demux/1
  Input_Select/1 -> Mux/1
  In4/1 -> Mux/2
  In5/1 -> Mux/3
  In6/1 -> Mux/4
  In7/1 -> Mux/5
  Mux/1 -> MAC PE/2(a_ij)
  x/1 -> MAC PE/1(x_i)
  MAC PE/1(y_1) -> Demux/2

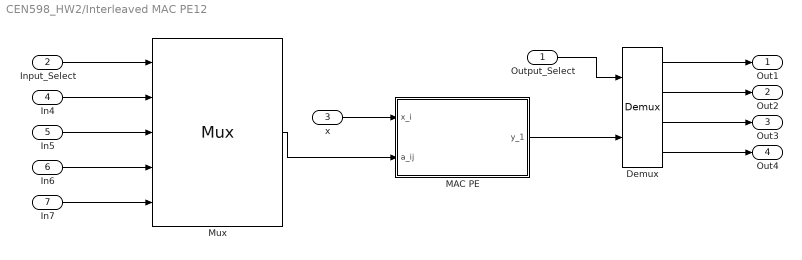
== system CEN598_HW2/Interleaved MAC PE12 ==
  Output_Select : Inport
  Input_Select : Inport  Port=2
  x : Inport  Port=3
  In4 : Inport  Port=4
  In5 : Inport  Port=5
  In6 : Inport  Port=6
  In7 : Inport  Port=7
  Demux : shlslibv1/Signal Operations/Demux  syn_out_nb=4  syn_out_latch=off  synBlockType=primitive  synLatency=0  synBlockId=18
  MAC PE : Subsystem
  Mux : shlslibv1/Signal Operations/Mux  syn_in_nb=4  syn_out_f=Full Precision  syn_out_wl=16  syn_out_fl=8  syn_out_dt=signed  syn_en_se=off  synBlockType=primitive  synLatency=0  synBlockId=16
  Out1 : Outport
  Out2 : Outport  Port=2
  Out3 : Outport  Port=3
  Out4 : Outport  Port=4
  wires:
  Demux/1 -> Out1/1
  Demux/2 -> Out2/1
  Demux/3 -> Out3/1
  Demux/4 -> Out4/1
  Output_Select/1 -> Demux/1
  Input_Select/1 -> Mux/1
  In4/1 -> Mux/2
  In5/1 -> Mux/3
  In6/1 -> Mux/4
  In7/1 -> Mux/5
  Mux/1 -> MAC PE/2(a_ij)
  x/1 -> MAC PE/1(x_i)
  MAC PE/1(y_1) -> Demux/2

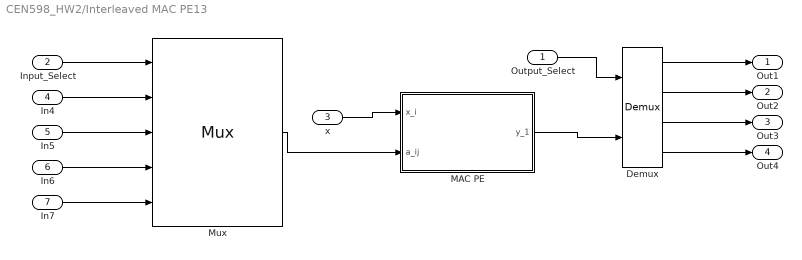
== system CEN598_HW2/Interleaved MAC PE13 ==
  Output_Select : Inport
  Input_Select : Inport  Port=2
  x : Inport  Port=3
  In4 : Inport  Port=4
  In5 : Inport  Port=5
  In6 : Inport  Port=6
  In7 : Inport  Port=7
  Demux : shlslibv1/Signal Operations/Demux  syn_out_nb=4  syn_out_latch=off  synBlockType=primitive  synLatency=0  synBlockId=18
  MAC PE : Subsystem
  Mux : shlslibv1/Signal Operations/Mux  syn_in_nb=4  syn_out_f=Full Precision  syn_out_wl=16  syn_out_fl=8  syn_out_dt=signed  syn_en_se=off  synBlockType=primitive  synLatency=0  synBlockId=16
  Out1 : Outport
  Out2 : Outport  Port=2
  Out3 : Outport  Port=3
  Out4 : Outport  Port=4
  wires:
  Demux/1 -> Out1/1
  Demux/2 -> Out2/1
  Demux/3 -> Out3/1
  Demux/4 -> Out4/1
  Output_Select/1 -> Demux/1
  Input_Select/1 -> Mux/1
  In4/1 -> Mux/2
  In5/1 -> Mux/3
  In6/1 -> Mux/4
  In7/1 -> Mux/5
  Mux/1 -> MAC PE/2(a_ij)
  x/1 -> MAC PE/1(x_i)
  MAC PE/1(y_1) -> Demux/2

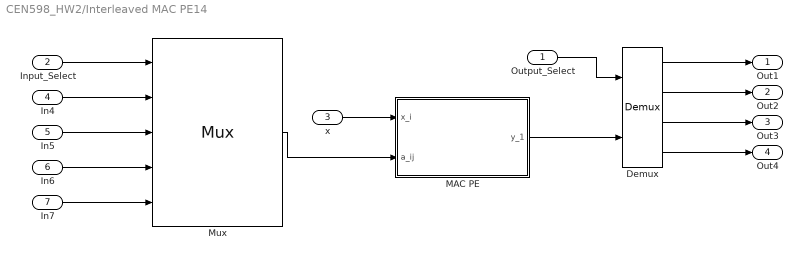
== system CEN598_HW2/Interleaved MAC PE14 ==
  Output_Select : Inport
  Input_Select : Inport  Port=2
  x : Inport  Port=3
  In4 : Inport  Port=4
  In5 : Inport  Port=5
  In6 : Inport  Port=6
  In7 : Inport  Port=7
  Demux : shlslibv1/Signal Operations/Demux  syn_out_nb=4  syn_out_latch=off  synBlockType=primitive  synLatency=0  synBlockId=18
  MAC PE : Subsystem
  Mux : shlslibv1/Signal Operations/Mux  syn_in_nb=4  syn_out_f=Full Precision  syn_out_wl=16  syn_out_fl=8  syn_out_dt=signed  syn_en_se=off  synBlockType=primitive  synLatency=0  synBlockId=16
  Out1 : Outport
  Out2 : Outport  Port=2
  Out3 : Outport  Port=3
  Out4 : Outport  Port=4
  wires:
  Demux/1 -> Out1/1
  Demux/2 -> Out2/1
  Demux/3 -> Out3/1
  Demux/4 -> Out4/1
  Output_Select/1 -> Demux/1
  Input_Select/1 -> Mux/1
  In4/1 -> Mux/2
  In5/1 -> Mux/3
  In6/1 -> Mux/4
  In7/1 -> Mux/5
  Mux/1 -> MAC PE/2(a_ij)
  x/1 -> MAC PE/1(x_i)
  MAC PE/1(y_1) -> Demux/2

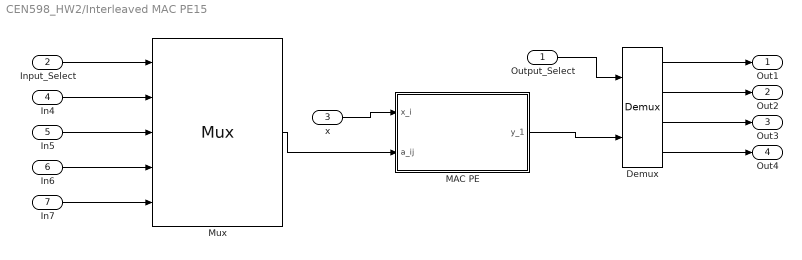
== system CEN598_HW2/Interleaved MAC PE15 ==
  Output_Select : Inport
  Input_Select : Inport  Port=2
  x : Inport  Port=3
  In4 : Inport  Port=4
  In5 : Inport  Port=5
  In6 : Inport  Port=6
  In7 : Inport  Port=7
  Demux : shlslibv1/Signal Operations/Demux  syn_out_nb=4  syn_out_latch=off  synBlockType=primitive  synLatency=0  synBlockId=18
  MAC PE : Subsystem
  Mux : shlslibv1/Signal Operations/Mux  syn_in_nb=4  syn_out_f=Full Precision  syn_out_wl=16  syn_out_fl=8  syn_out_dt=signed  syn_en_se=off  synBlockType=primitive  synLatency=0  synBlockId=16
  Out1 : Outport
  Out2 : Outport  Port=2
  Out3 : Outport  Port=3
  Out4 : Outport  Port=4
  wires:
  Demux/1 -> Out1/1
  Demux/2 -> Out2/1
  Demux/3 -> Out3/1
  Demux/4 -> Out4/1
  Output_Select/1 -> Demux/1
  Input_Select/1 -> Mux/1
  In4/1 -> Mux/2
  In5/1 -> Mux/3
  In6/1 -> Mux/4
  In7/1 -> Mux/5
  Mux/1 -> MAC PE/2(a_ij)
  x/1 -> MAC PE/1(x_i)
  MAC PE/1(y_1) -> Demux/2

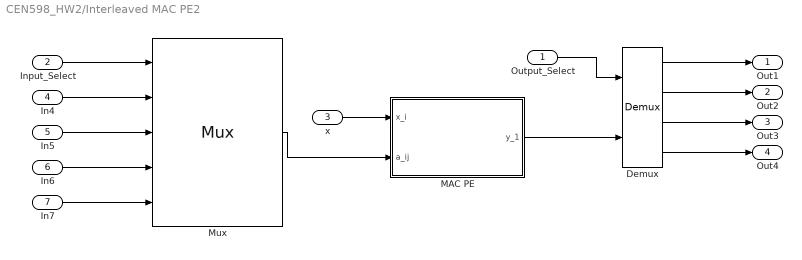
== system CEN598_HW2/Interleaved MAC PE2 ==
  Output_Select : Inport
  Input_Select : Inport  Port=2
  x : Inport  Port=3
  In4 : Inport  Port=4
  In5 : Inport  Port=5
  In6 : Inport  Port=6
  In7 : Inport  Port=7
  Demux : shlslibv1/Signal Operations/Demux  syn_out_nb=4  syn_out_latch=off  synBlockType=primitive  synLatency=0  synBlockId=18
  MAC PE : Subsystem
  Mux : shlslibv1/Signal Operations/Mux  syn_in_nb=4  syn_out_f=Full Precision  syn_out_wl=16  syn_out_fl=8  syn_out_dt=signed  syn_en_se=off  synBlockType=primitive  synLatency=0  synBlockId=16
  Out1 : Outport
  Out2 : Outport  Port=2
  Out3 : Outport  Port=3
  Out4 : Outport  Port=4
  wires:
  Demux/1 -> Out1/1
  Demux/2 -> Out2/1
  Demux/3 -> Out3/1
  Demux/4 -> Out4/1
  Output_Select/1 -> Demux/1
  Input_Select/1 -> Mux/1
  In4/1 -> Mux/2
  In5/1 -> Mux/3
  In6/1 -> Mux/4
  In7/1 -> Mux/5
  Mux/1 -> MAC PE/2(a_ij)
  x/1 -> MAC PE/1(x_i)
  MAC PE/1(y_1) -> Demux/2

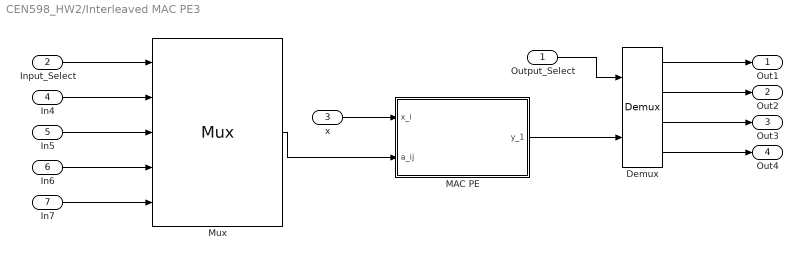
== system CEN598_HW2/Interleaved MAC PE3 ==
  Output_Select : Inport
  Input_Select : Inport  Port=2
  x : Inport  Port=3
  In4 : Inport  Port=4
  In5 : Inport  Port=5
  In6 : Inport  Port=6
  In7 : Inport  Port=7
  Demux : shlslibv1/Signal Operations/Demux  syn_out_nb=4  syn_out_latch=off  synBlockType=primitive  synLatency=0  synBlockId=18
  MAC PE : Subsystem
  Mux : shlslibv1/Signal Operations/Mux  syn_in_nb=4  syn_out_f=Full Precision  syn_out_wl=16  syn_out_fl=8  syn_out_dt=signed  syn_en_se=off  synBlockType=primitive  synLatency=0  synBlockId=16
  Out1 : Outport
  Out2 : Outport  Port=2
  Out3 : Outport  Port=3
  Out4 : Outport  Port=4
  wires:
  Demux/1 -> Out1/1
  Demux/2 -> Out2/1
  Demux/3 -> Out3/1
  Demux/4 -> Out4/1
  Output_Select/1 -> Demux/1
  Input_Select/1 -> Mux/1
  In4/1 -> Mux/2
  In5/1 -> Mux/3
  In6/1 -> Mux/4
  In7/1 -> Mux/5
  Mux/1 -> MAC PE/2(a_ij)
  x/1 -> MAC PE/1(x_i)
  MAC PE/1(y_1) -> Demux/2

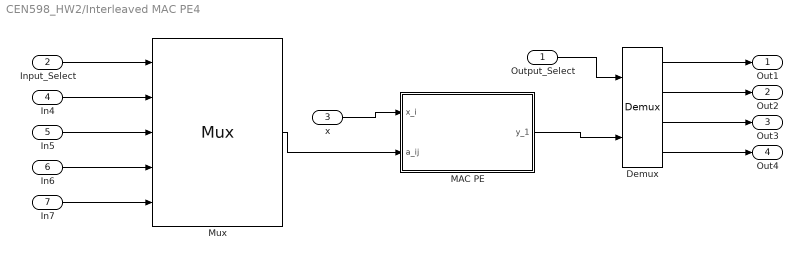
== system CEN598_HW2/Interleaved MAC PE4 ==
  Output_Select : Inport
  Input_Select : Inport  Port=2
  x : Inport  Port=3
  In4 : Inport  Port=4
  In5 : Inport  Port=5
  In6 : Inport  Port=6
  In7 : Inport  Port=7
  Demux : shlslibv1/Signal Operations/Demux  syn_out_nb=4  syn_out_latch=off  synBlockType=primitive  synLatency=0  synBlockId=18
  MAC PE : Subsystem
  Mux : shlslibv1/Signal Operations/Mux  syn_in_nb=4  syn_out_f=Full Precision  syn_out_wl=16  syn_out_fl=8  syn_out_dt=signed  syn_en_se=off  synBlockType=primitive  synLatency=0  synBlockId=16
  Out1 : Outport
  Out2 : Outport  Port=2
  Out3 : Outport  Port=3
  Out4 : Outport  Port=4
  wires:
  Demux/1 -> Out1/1
  Demux/2 -> Out2/1
  Demux/3 -> Out3/1
  Demux/4 -> Out4/1
  Output_Select/1 -> Demux/1
  Input_Select/1 -> Mux/1
  In4/1 -> Mux/2
  In5/1 -> Mux/3
  In6/1 -> Mux/4
  In7/1 -> Mux/5
  Mux/1 -> MAC PE/2(a_ij)
  x/1 -> MAC PE/1(x_i)
  MAC PE/1(y_1) -> Demux/2

== system CEN598_HW2/Interleaved MAC PE5 ==
  Output_Select : Inport
  Input_Select : Inport  Port=2
  x : Inport  Port=3
  In4 : Inport  Port=4
  In5 : Inport  Port=5
  In6 : Inport  Port=6
  In7 : Inport  Port=7
  Demux : shlslibv1/Signal Operations/Demux  syn_out_nb=4  syn_out_latch=off  synBlockType=primitive  synLatency=0  synBlockId=18
  MAC PE : Subsystem
  Mux : shlslibv1/Signal Operations/Mux  syn_in_nb=4  syn_out_f=Full Precision  syn_out_wl=16  syn_out_fl=8  syn_out_dt=signed  syn_en_se=off  synBlockType=primitive  synLatency=0  synBlockId=16
  Out1 : Outport
  Out2 : Outport  Port=2
  Out3 : Outport  Port=3
  Out4 : Outport  Port=4
  wires:
  Demux/1 -> Out1/1
  Demux/2 -> Out2/1
  Demux/3 -> Out3/1
  Demux/4 -> Out4/1
  Output_Select/1 -> Demux/1
  Input_Select/1 -> Mux/1
  In4/1 -> Mux/2
  In5/1 -> Mux/3
  In6/1 -> Mux/4
  In7/1 -> Mux/5
  Mux/1 -> MAC PE/2(a_ij)
  x/1 -> MAC PE/1(x_i)
  MAC PE/1(y_1) -> Demux/2

== system CEN598_HW2/Interleaved MAC PE6 ==
  Output_Select : Inport
  Input_Select : Inport  Port=2
  x : Inport  Port=3
  In4 : Inport  Port=4
  In5 : Inport  Port=5
  In6 : Inport  Port=6
  In7 : Inport  Port=7
  Demux : shlslibv1/Signal Operations/Demux  syn_out_nb=4  syn_out_latch=off  synBlockType=primitive  synLatency=0  synBlockId=18
  MAC PE : Subsystem
  Mux : shlslibv1/Signal Operations/Mux  syn_in_nb=4  syn_out_f=Full Precision  syn_out_wl=16  syn_out_fl=8  syn_out_dt=signed  syn_en_se=off  synBlockType=primitive  synLatency=0  synBlockId=16
  Out1 : Outport
  Out2 : Outport  Port=2
  Out3 : Outport  Port=3
  Out4 : Outport  Port=4
  wires:
  Demux/1 -> Out1/1
  Demux/2 -> Out2/1
  Demux/3 -> Out3/1
  Demux/4 -> Out4/1
  Output_Select/1 -> Demux/1
  Input_Select/1 -> Mux/1
  In4/1 -> Mux/2
  In5/1 -> Mux/3
  In6/1 -> Mux/4
  In7/1 -> Mux/5
  Mux/1 -> MAC PE/2(a_ij)
  x/1 -> MAC PE/1(x_i)
  MAC PE/1(y_1) -> Demux/2

== system CEN598_HW2/Interleaved MAC PE7 ==
  Output_Select : Inport
  Input_Select : Inport  Port=2
  x : Inport  Port=3
  In4 : Inport  Port=4
  In5 : Inport  Port=5
  In6 : Inport  Port=6
  In7 : Inport  Port=7
  Demux : shlslibv1/Signal Operations/Demux  syn_out_nb=4  syn_out_latch=off  synBlockType=primitive  synLatency=0  synBlockId=18
  MAC PE : Subsystem
  Mux : shlslibv1/Signal Operations/Mux  syn_in_nb=4  syn_out_f=Full Precision  syn_out_wl=16  syn_out_fl=8  syn_out_dt=signed  syn_en_se=off  synBlockType=primitive  synLatency=0  synBlockId=16
  Out1 : Outport
  Out2 : Outport  Port=2
  Out3 : Outport  Port=3
  Out4 : Outport  Port=4
  wires:
  Demux/1 -> Out1/1
  Demux/2 -> Out2/1
  Demux/3 -> Out3/1
  Demux/4 -> Out4/1
  Output_Select/1 -> Demux/1
  Input_Select/1 -> Mux/1
  In4/1 -> Mux/2
  In5/1 -> Mux/3
  In6/1 -> Mux/4
  In7/1 -> Mux/5
  Mux/1 -> MAC PE/2(a_ij)
  x/1 -> MAC PE/1(x_i)
  MAC PE/1(y_1) -> Demux/2

== system CEN598_HW2/Interleaved MAC PE8 ==
  Output_Select : Inport
  Input_Select : Inport  Port=2
  x : Inport  Port=3
  In4 : Inport  Port=4
  In5 : Inport  Port=5
  In6 : Inport  Port=6
  In7 : Inport  Port=7
  Demux : shlslibv1/Signal Operations/Demux  syn_out_nb=4  syn_out_latch=off  synBlockType=primitive  synLatency=0  synBlockId=18
  MAC PE : Subsystem
  Mux : shlslibv1/Signal Operations/Mux  syn_in_nb=4  syn_out_f=Full Precision  syn_out_wl=16  syn_out_fl=8  syn_out_dt=signed  syn_en_se=off  synBlockType=primitive  synLatency=0  synBlockId=16
  Out1 : Outport
  Out2 : Outport  Port=2
  Out3 : Outport  Port=3
  Out4 : Outport  Port=4
  wires:
  Demux/1 -> Out1/1
  Demux/2 -> Out2/1
  Demux/3 -> Out3/1
  Demux/4 -> Out4/1
  Output_Select/1 -> Demux/1
  Input_Select/1 -> Mux/1
  In4/1 -> Mux/2
  In5/1 -> Mux/3
  In6/1 -> Mux/4
  In7/1 -> Mux/5
  Mux/1 -> MAC PE/2(a_ij)
  x/1 -> MAC PE/1(x_i)
  MAC PE/1(y_1) -> Demux/2

== system CEN598_HW2/Interleaved MAC PE9 ==
  Output_Select : Inport
  Input_Select : Inport  Port=2
  x : Inport  Port=3
  In4 : Inport  Port=4
  In5 : Inport  Port=5
  In6 : Inport  Port=6
  In7 : Inport  Port=7
  Demux : shlslibv1/Signal Operations/Demux  syn_out_nb=4  syn_out_latch=off  synBlockType=primitive  synLatency=0  synBlockId=18
  MAC PE : Subsystem
  Mux : shlslibv1/Signal Operations/Mux  syn_in_nb=4  syn_out_f=Full Precision  syn_out_wl=16  syn_out_fl=8  syn_out_dt=signed  syn_en_se=off  synBlockType=primitive  synLatency=0  synBlockId=16
  Out1 : Outport
  Out2 : Outport  Port=2
  Out3 : Outport  Port=3
  Out4 : Outport  Port=4
  wires:
  Demux/1 -> Out1/1
  Demux/2 -> Out2/1
  Demux/3 -> Out3/1
  Demux/4 -> Out4/1
  Output_Select/1 -> Demux/1
  Input_Select/1 -> Mux/1
  In4/1 -> Mux/2
  In5/1 -> Mux/3
  In6/1 -> Mux/4
  In7/1 -> Mux/5
  Mux/1 -> MAC PE/2(a_ij)
  x/1 -> MAC PE/1(x_i)
  MAC PE/1(y_1) -> Demux/2

== system CEN598_HW2/Interleaved MAC PE/MAC PE ==
  x_i : Inport
  a_ij : Inport  Port=2
  FP Add : shlslibv1/Floating Point/FP Add  syn_exp_wl=11  syn_frac_wl=52  syn_opt_ports=off  syn_add_opr=add  synBlockType=custom  synLatency=9
  FP Constant : shlslibv1/Floating Point/FP Constant  syn_constant_val=1  syn_exp_wl=11  syn_frac_wl=52  syn_cst_st=1/284.04e6  synBlockType=custom  synLatency=0
  FP Mult : shlslibv1/Floating Point/FP Mult  syn_exp_wl=11  syn_frac_wl=52  syn_opt_ports=off  synBlockType=custom  synLatency=3  syn_opt_tar=Default  syn_fracmult_pipe=1
  Terminator : Terminator
  y_1 : Outport
  wires:
  x_i/1 -> FP Mult/1
  a_ij/1 -> FP Mult/2
  FP Mult/1 -> FP Add/2
  FP Mult/2 -> FP Add/3
  FP Add/1 -> FP Add/1, y_1/1
  FP Add/2 -> Terminator/1
  FP Constant/1 -> FP Mult/3

== system CEN598_HW2/Interleaved MAC PE1/MAC PE ==
  x_i : Inport
  a_ij : Inport  Port=2
  FP Add : shlslibv1/Floating Point/FP Add  syn_exp_wl=11  syn_frac_wl=52  syn_opt_ports=off  syn_add_opr=add  synBlockType=custom  synLatency=9
  FP Constant : shlslibv1/Floating Point/FP Constant  syn_constant_val=1  syn_exp_wl=11  syn_frac_wl=52  syn_cst_st=1/284.04e6  synBlockType=custom  synLatency=0
  FP Mult : shlslibv1/Floating Point/FP Mult  syn_exp_wl=11  syn_frac_wl=52  syn_opt_ports=off  synBlockType=custom  synLatency=3  syn_opt_tar=Default  syn_fracmult_pipe=1
  Terminator : Terminator
  y_1 : Outport
  wires:
  x_i/1 -> FP Mult/1
  a_ij/1 -> FP Mult/2
  FP Mult/1 -> FP Add/2
  FP Mult/2 -> FP Add/3
  FP Add/1 -> FP Add/1, y_1/1
  FP Add/2 -> Terminator/1
  FP Constant/1 -> FP Mult/3

== system CEN598_HW2/Interleaved MAC PE10/MAC PE ==
  x_i : Inport
  a_ij : Inport  Port=2
  FP Add : shlslibv1/Floating Point/FP Add  syn_exp_wl=11  syn_frac_wl=52  syn_opt_ports=off  syn_add_opr=add  synBlockType=custom  synLatency=9
  FP Constant : shlslibv1/Floating Point/FP Constant  syn_constant_val=1  syn_exp_wl=11  syn_frac_wl=52  syn_cst_st=1/284.04e6  synBlockType=custom  synLatency=0
  FP Mult : shlslibv1/Floating Point/FP Mult  syn_exp_wl=11  syn_frac_wl=52  syn_opt_ports=off  synBlockType=custom  synLatency=3  syn_opt_tar=Default  syn_fracmult_pipe=1
  Terminator : Terminator
  y_1 : Outport
  wires:
  x_i/1 -> FP Mult/1
  a_ij/1 -> FP Mult/2
  FP Mult/1 -> FP Add/2
  FP Mult/2 -> FP Add/3
  FP Add/1 -> FP Add/1, y_1/1
  FP Add/2 -> Terminator/1
  FP Constant/1 -> FP Mult/3
